simulink model "mpc_weightsdemo"  (Simulink 6.5)
settings: Solver=ode45  SolverMode=SingleTasking  StartTime=0.0  StopTime=Tstop  RelTol=1e-3
values from neighbouring files (symbols this model uses):
  A = [-.0151 -60.5651 0 -32.174 ... (first row only)    [afti16.m]    (also in mpcutarget.m = sys.a)
  B = [-2.516 -13.136 ... (first row only)    [afti16.m]    (also in mpcutarget.m = sys.b)
  C = [0 1 0 0 ... (first row only)    [afti16.m]    (also in mpcutarget.m = sys.c)
  D = [0 0 ... (first row only)    [afti16.m]    (also in mpccstr.m = ss(getindist(MPC)); mpcutarget.m = sys.d)
libraries: mpclib x1
settings Model: Creator=jowen  LastModifiedBy=Alberto Bemporad  ExtModeTrigMode=oneshot  ExtModeArmWhenConnect=off
settings DataIOCC: LimitDataPoints=off  SignalLoggingName=sigsOut
settings OptimizationCC: BooleanDataType=off  InlineInvariantSignals=on
settings DebuggingCC: CheckExecutionContextPreStartOutputMsg=on  CheckExecutionContextRuntimeOutputMsg=on  SolverPrmCheckMsg=none  MultiTaskDSMMsg=warning  MultiTaskCondExecSysMsg=none  IntegerOverflowMsg=none  StrictBusMsg=None
settings HardwareCC: TargetUnknown=on
settings RTWCC: IncludeERTFirstTime=on

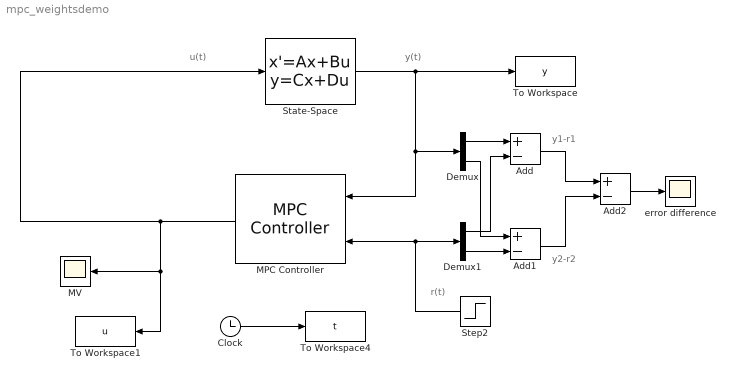
== system mpc_weightsdemo ==
  note: u(t)
  note: y(t)
  note: r(t)
  note: y1-r1
  note: y2-r2
  Add : Sum  Inputs=+-  OutScaling=2^-10
  Add1 : Sum  Inputs=+-  OutScaling=2^-10
  Add2 : Sum  Inputs=+-  OutScaling=2^-10
  Clock : Clock
      settings: Decimation=10
  Demux : Demux  Outputs=2
  Demux1 : Demux  Outputs=2
  MPC Controller : mpclib/MPC Controller  Orientation=left  SystemSampleTime=-1  mpcobj=MPCobj  n_mv=0  x0=[]  ref_from_ws=off  ref_signal_name=[]  ref_preview=on  md_from_ws=off  md_signal_name=[]  md_preview=on  from_project=off  md_inport=off  mv_inport=off  lims_inport=off  project_file=MPCtask.mat
  MV : Scope
      settings: TimeRange=30  YMin=-3  YMax=2  DataFormat=Structure
  State-Space : StateSpace  A=A  B=B  C=C  D=D  X0=[0 0 0 0 0 0 0]'
  Step2 : Step  Orientation=left  Time=0  After=[1 2]  SampleTime=0
  To Workspace : ToWorkspace  VariableName=y  SampleTime=-1  SaveFormat=Array
      settings: MaxDataPoints=Inf
  To Workspace1 : ToWorkspace  VariableName=u  SampleTime=-1  SaveFormat=Array
      settings: MaxDataPoints=Inf
  To Workspace4 : ToWorkspace  VariableName=t  SampleTime=-1  SaveFormat=Array
      settings: MaxDataPoints=Inf
  error difference : Scope
      settings: TimeRange=30  YMin=-0.5  YMax=1  DataFormat=Structure
  wires:
  Step2/1 -> MPC Controller/2, Demux1/1
  State-Space/1 -> To Workspace/1, MPC Controller/1, Demux/1
  MPC Controller/1 -> MV/1, To Workspace1/1, State-Space/1
  Clock/1 -> To Workspace4/1
  Demux/1 -> Add/1
  Demux1/1 -> Add/2
  Demux/2 -> Add1/1
  Demux1/2 -> Add1/2
  Add/1 -> Add2/1
  Add1/1 -> Add2/2
  Add2/1 -> error difference/1
